simulink model "b_2x_8a_r308d"  (Simulink 6.2)
settings: Solver=ode45  StartTime=0.0  StopTime=1030.0  RelTol=1e-3
undefined symbols (not defined in the file): ant_bits, BEE2_usr, blockCountBits, blockRowBits, cmult_4bit_em
libraries: xbsIndex_r3 x3300, xps_library x102, casper_library x97
(part 5 of 22)

== system b_2x_8a_r308d/snap_gbe_tx ==
  data_in : Inport  Port=1  LatchInput=off
  oob_in : Inport  Port=2  LatchInput=off
  trig : Inport  Port=3  LatchInput=off
  we : Inport  Port=4  LatchInput=off
  Constant : xbsIndex_r3/Constant  const=1  equ=P=C  arith_type=Boolean  n_bits=1  bin_pt=0  opselect=C  inp2=PCIN>>17  opr=+  inp1=P  carry=CIN  iostate=0  explicit_period=on  period=1  dbl_ovrd=off
  Constant1 : xbsIndex_r3/Constant  const=1  equ=P=C  arith_type=Boolean  n_bits=1  bin_pt=0  opselect=C  inp2=PCIN>>17  opr=+  inp1=P  carry=CIN  iostate=0  explicit_period=on  period=1  dbl_ovrd=off
  Constant13 : Constant
  Constant2 : xbsIndex_r3/Constant  const=1  equ=P=C  arith_type=Boolean  n_bits=1  bin_pt=0  opselect=C  inp2=PCIN>>17  opr=+  inp1=P  carry=CIN  iostate=0  explicit_period=on  period=1  dbl_ovrd=off
  Inverter : xbsIndex_r3/Inverter  latency=0  explicit_period=off  period=1  en=off  dbl_ovrd=off  show_param=off
      settings: xl_area=[0, 0, 0, 0, 0, 0, 0]
  Logical1 : xbsIndex_r3/Logical  logical_function=AND  inputs=2  precision=Full  arith_type=Unsigned  n_bits=8  bin_pt=2  align_bp=on  latency=0  explicit_period=off  period=1  en=off  dbl_ovrd=off  show_param=off
      settings: xl_area=[0, 0, 0, 0, 0, 0, 0]
  Mux1 : xbsIndex_r3/Mux  inputs=2  precision=Full  arith_type="Signed  (2's comp)"  n_bits=8  bin_pt=2  quantization=Truncate  overflow=Wrap  latency=0  explicit_period=off  period=1  en=off  dbl_ovrd=off  show_param=off  mux_type=off  use_rpm=off  gen_core=off
      settings: xl_area=[0, 0, 0, 0, 0, 0, 0]
  Mux2 : xbsIndex_r3/Mux  inputs=2  precision=Full  arith_type="Signed  (2's comp)"  n_bits=8  bin_pt=2  quantization=Truncate  overflow=Wrap  latency=0  explicit_period=off  period=1  en=off  dbl_ovrd=off  show_param=off  mux_type=off  use_rpm=off  gen_core=off
      settings: xl_area=[0, 0, 0, 0, 0, 0, 0]
  Register : xbsIndex_r3/Register  init=0  reg_only_valid=off  explicit_period=off  period=1  rst=on  en=on  out_en=off  dbl_ovrd=off  show_param=off
      settings: xl_area=[0, 0, 0, 0, 0, 0, 0]
  Register1 : xbsIndex_r3/Register  init=0  reg_only_valid=off  explicit_period=off  period=1  rst=on  en=on  out_en=off  dbl_ovrd=off  show_param=off
      settings: xl_area=[0, 0, 0, 0, 0, 0, 0]
  Reinterpret3 : xbsIndex_r3/Reinterpret  force_arith_type=on  arith_type=Unsigned  force_bin_pt=on  bin_pt=0  force_valid=on
  addr : xps_library/software register  Tag=xps:sw_reg  io_dir=To Processor  arith_type=Unsigned  bitwidth=32  bin_pt=0  sample_period=1  gw_name=b_2x_8a_r308d_snap_gbe_tx_addr_user_data_in
  bram_lsb : xps_library/Shared BRAM  Tag=xps:bram  arith_type=Unsigned  addr_width=nsamples  data_width=32  data_bin_pt=0  init_vals=0  sample_rate=1
  bram_msb : xps_library/Shared BRAM  Tag=xps:bram  arith_type=Unsigned  addr_width=nsamples  data_width=32  data_bin_pt=0  init_vals=0  sample_rate=1
  bram_oob : xps_library/Shared BRAM  Tag=xps:bram  arith_type=Unsigned  addr_width=nsamples  data_width=32  data_bin_pt=0  init_vals=0  sample_rate=1
  ctrl : xps_library/software register  Tag=xps:sw_reg  io_dir=From Processor  arith_type=Unsigned  bitwidth=32  bin_pt=0  sample_period=1  gw_name=b_2x_8a_r308d_snap_gbe_tx_ctrl_user_data_out
  en1 : xbsIndex_r3/Slice  mode=Lower Bit Location + Width  nbits=32  bit1=0  base1=LSB of Input  bit0=32  base0=LSB of Input  boolean_output=off  explicit_period=off  period=1  dbl_ovrd=off
  en2 : xbsIndex_r3/Slice  mode=Lower Bit Location + Width  nbits=32  bit1=0  base1=LSB of Input  bit0=0  base0=LSB of Input  boolean_output=off  explicit_period=off  period=1  dbl_ovrd=off
  enable : xbsIndex_r3/Slice  mode=Lower Bit Location + Width  nbits=1  bit1=0  base1=LSB of Input  bit0=0  base0=LSB of Input  boolean_output=on  explicit_period=off  period=1  dbl_ovrd=off
  freeze_cntr : casper_library/Misc/freeze_cntr  CounterBits=nsamples
  posedge : casper_library/Misc/posedge  Tag=Rising Edge Detector
  trig1 : xbsIndex_r3/Slice  mode=Lower Bit Location + Width  nbits=1  bit1=0  base1=LSB of Input  bit0=1  base0=LSB of Input  boolean_output=on  explicit_period=off  period=1  dbl_ovrd=off
  valid : xbsIndex_r3/Slice  mode=Lower Bit Location + Width  nbits=1  bit1=0  base1=LSB of Input  bit0=2  base0=LSB of Input  boolean_output=on  explicit_period=off  period=1  dbl_ovrd=off
  wires:
  freeze_cntr/1 -> bram_lsb/1, bram_msb/1, bram_oob/1, Register1/1
  Register/1 -> freeze_cntr/2
  Mux2/1 -> Logical1/1
  Inverter/1 -> Logical1/2
  Logical1/1 -> Register/2
  valid/1 -> Mux1/1
  trig1/1 -> Mux2/1
  Register1/1 -> addr/1
  Constant2/1 -> Mux1/3
  we/1 -> Mux1/2
  Mux1/1 -> freeze_cntr/1
  Constant1/1 -> Mux2/3
  Constant/1 -> Register/1
  posedge/1 -> Inverter/1, Register1/2, Register/3
  ctrl/1 -> trig1/1, valid/1, enable/1
  Constant13/1 -> ctrl/1
  freeze_cntr/2 -> bram_lsb/3, bram_msb/3, bram_oob/3, Register1/3
  enable/1 -> posedge/1
  trig/1 -> Mux2/2
  Reinterpret3/1 -> en1/1, en2/1
  data_in/1 -> Reinterpret3/1
  en1/1 -> bram_msb/2
  en2/1 -> bram_lsb/2
  oob_in/1 -> bram_oob/2

== system b_2x_8a_r308d/snap_rx ==
  data_in : Inport  Port=1  LatchInput=off
  oob_in : Inport  Port=2  LatchInput=off
  trig : Inport  Port=3  LatchInput=off
  we : Inport  Port=4  LatchInput=off
  Constant : xbsIndex_r3/Constant  const=1  equ=P=C  arith_type=Boolean  n_bits=1  bin_pt=0  opselect=C  inp2=PCIN>>17  opr=+  inp1=P  carry=CIN  iostate=0  explicit_period=on  period=1  dbl_ovrd=off
  Constant1 : xbsIndex_r3/Constant  const=1  equ=P=C  arith_type=Boolean  n_bits=1  bin_pt=0  opselect=C  inp2=PCIN>>17  opr=+  inp1=P  carry=CIN  iostate=0  explicit_period=on  period=1  dbl_ovrd=off
  Constant13 : Constant
  Constant2 : xbsIndex_r3/Constant  const=1  equ=P=C  arith_type=Boolean  n_bits=1  bin_pt=0  opselect=C  inp2=PCIN>>17  opr=+  inp1=P  carry=CIN  iostate=0  explicit_period=on  period=1  dbl_ovrd=off
  Inverter : xbsIndex_r3/Inverter  latency=0  explicit_period=off  period=1  en=off  dbl_ovrd=off  show_param=off
      settings: xl_area=[0, 0, 0, 0, 0, 0, 0]
  Logical1 : xbsIndex_r3/Logical  logical_function=AND  inputs=2  precision=Full  arith_type=Unsigned  n_bits=8  bin_pt=2  align_bp=on  latency=0  explicit_period=off  period=1  en=off  dbl_ovrd=off  show_param=off
      settings: xl_area=[0, 0, 0, 0, 0, 0, 0]
  Mux1 : xbsIndex_r3/Mux  inputs=2  precision=Full  arith_type="Signed  (2's comp)"  n_bits=8  bin_pt=2  quantization=Truncate  overflow=Wrap  latency=0  explicit_period=off  period=1  en=off  dbl_ovrd=off  show_param=off  mux_type=off  use_rpm=off  gen_core=off
      settings: xl_area=[0, 0, 0, 0, 0, 0, 0]
  Mux2 : xbsIndex_r3/Mux  inputs=2  precision=Full  arith_type="Signed  (2's comp)"  n_bits=8  bin_pt=2  quantization=Truncate  overflow=Wrap  latency=0  explicit_period=off  period=1  en=off  dbl_ovrd=off  show_param=off  mux_type=off  use_rpm=off  gen_core=off
      settings: xl_area=[0, 0, 0, 0, 0, 0, 0]
  Register : xbsIndex_r3/Register  init=0  reg_only_valid=off  explicit_period=off  period=1  rst=on  en=on  out_en=off  dbl_ovrd=off  show_param=off
      settings: xl_area=[0, 0, 0, 0, 0, 0, 0]
  Register1 : xbsIndex_r3/Register  init=0  reg_only_valid=off  explicit_period=off  period=1  rst=on  en=on  out_en=off  dbl_ovrd=off  show_param=off
      settings: xl_area=[0, 0, 0, 0, 0, 0, 0]
  Reinterpret3 : xbsIndex_r3/Reinterpret  force_arith_type=on  arith_type=Unsigned  force_bin_pt=on  bin_pt=0  force_valid=on
  addr : xps_library/software register  Tag=xps:sw_reg  io_dir=To Processor  arith_type=Unsigned  bitwidth=32  bin_pt=0  sample_period=1  gw_name=b_2x_8a_r308d_snap_rx_addr_user_data_in
  bram_lsb : xps_library/Shared BRAM  Tag=xps:bram  arith_type=Unsigned  addr_width=nsamples  data_width=32  data_bin_pt=0  init_vals=0  sample_rate=1
  bram_msb : xps_library/Shared BRAM  Tag=xps:bram  arith_type=Unsigned  addr_width=nsamples  data_width=32  data_bin_pt=0  init_vals=0  sample_rate=1
  bram_oob : xps_library/Shared BRAM  Tag=xps:bram  arith_type=Unsigned  addr_width=nsamples  data_width=32  data_bin_pt=0  init_vals=0  sample_rate=1
  ctrl : xps_library/software register  Tag=xps:sw_reg  io_dir=From Processor  arith_type=Unsigned  bitwidth=32  bin_pt=0  sample_period=1  gw_name=b_2x_8a_r308d_snap_rx_ctrl_user_data_out
  en1 : xbsIndex_r3/Slice  mode=Lower Bit Location + Width  nbits=32  bit1=0  base1=LSB of Input  bit0=32  base0=LSB of Input  boolean_output=off  explicit_period=off  period=1  dbl_ovrd=off
  en2 : xbsIndex_r3/Slice  mode=Lower Bit Location + Width  nbits=32  bit1=0  base1=LSB of Input  bit0=0  base0=LSB of Input  boolean_output=off  explicit_period=off  period=1  dbl_ovrd=off
  enable : xbsIndex_r3/Slice  mode=Lower Bit Location + Width  nbits=1  bit1=0  base1=LSB of Input  bit0=0  base0=LSB of Input  boolean_output=on  explicit_period=off  period=1  dbl_ovrd=off
  freeze_cntr : casper_library/Misc/freeze_cntr  CounterBits=nsamples
  posedge : casper_library/Misc/posedge  Tag=Rising Edge Detector
  trig1 : xbsIndex_r3/Slice  mode=Lower Bit Location + Width  nbits=1  bit1=0  base1=LSB of Input  bit0=1  base0=LSB of Input  boolean_output=on  explicit_period=off  period=1  dbl_ovrd=off
  valid : xbsIndex_r3/Slice  mode=Lower Bit Location + Width  nbits=1  bit1=0  base1=LSB of Input  bit0=2  base0=LSB of Input  boolean_output=on  explicit_period=off  period=1  dbl_ovrd=off
  wires:
  freeze_cntr/1 -> bram_lsb/1, bram_msb/1, bram_oob/1, Register1/1
  Register/1 -> freeze_cntr/2
  Mux2/1 -> Logical1/1
  Inverter/1 -> Logical1/2
  Logical1/1 -> Register/2
  valid/1 -> Mux1/1
  trig1/1 -> Mux2/1
  Register1/1 -> addr/1
  Constant2/1 -> Mux1/3
  we/1 -> Mux1/2
  Mux1/1 -> freeze_cntr/1
  Constant1/1 -> Mux2/3
  Constant/1 -> Register/1
  posedge/1 -> Inverter/1, Register1/2, Register/3
  ctrl/1 -> trig1/1, valid/1, enable/1
  Constant13/1 -> ctrl/1
  freeze_cntr/2 -> bram_lsb/3, bram_msb/3, bram_oob/3, Register1/3
  enable/1 -> posedge/1
  trig/1 -> Mux2/2
  Reinterpret3/1 -> en1/1, en2/1
  data_in/1 -> Reinterpret3/1
  en1/1 -> bram_msb/2
  en2/1 -> bram_lsb/2
  oob_in/1 -> bram_oob/2

== system b_2x_8a_r308d/snap_xaui ==
  data_in : Inport  Port=1  LatchInput=off
  oob_in : Inport  Port=2  LatchInput=off
  trig : Inport  Port=3  LatchInput=off
  we : Inport  Port=4  LatchInput=off
  Constant : xbsIndex_r3/Constant  const=1  equ=P=C  arith_type=Boolean  n_bits=1  bin_pt=0  opselect=C  inp2=PCIN>>17  opr=+  inp1=P  carry=CIN  iostate=0  explicit_period=on  period=1  dbl_ovrd=off
  Constant1 : xbsIndex_r3/Constant  const=1  equ=P=C  arith_type=Boolean  n_bits=1  bin_pt=0  opselect=C  inp2=PCIN>>17  opr=+  inp1=P  carry=CIN  iostate=0  explicit_period=on  period=1  dbl_ovrd=off
  Constant13 : Constant
  Constant2 : xbsIndex_r3/Constant  const=1  equ=P=C  arith_type=Boolean  n_bits=1  bin_pt=0  opselect=C  inp2=PCIN>>17  opr=+  inp1=P  carry=CIN  iostate=0  explicit_period=on  period=1  dbl_ovrd=off
  Inverter : xbsIndex_r3/Inverter  latency=0  explicit_period=off  period=1  en=off  dbl_ovrd=off  show_param=off
      settings: xl_area=[0, 0, 0, 0, 0, 0, 0]
  Logical1 : xbsIndex_r3/Logical  logical_function=AND  inputs=2  precision=Full  arith_type=Unsigned  n_bits=8  bin_pt=2  align_bp=on  latency=0  explicit_period=off  period=1  en=off  dbl_ovrd=off  show_param=off
      settings: xl_area=[0, 0, 0, 0, 0, 0, 0]
  Mux1 : xbsIndex_r3/Mux  inputs=2  precision=Full  arith_type="Signed  (2's comp)"  n_bits=8  bin_pt=2  quantization=Truncate  overflow=Wrap  latency=0  explicit_period=off  period=1  en=off  dbl_ovrd=off  show_param=off  mux_type=off  use_rpm=off  gen_core=off
      settings: xl_area=[0, 0, 0, 0, 0, 0, 0]
  Mux2 : xbsIndex_r3/Mux  inputs=2  precision=Full  arith_type="Signed  (2's comp)"  n_bits=8  bin_pt=2  quantization=Truncate  overflow=Wrap  latency=0  explicit_period=off  period=1  en=off  dbl_ovrd=off  show_param=off  mux_type=off  use_rpm=off  gen_core=off
      settings: xl_area=[0, 0, 0, 0, 0, 0, 0]
  Register : xbsIndex_r3/Register  init=0  reg_only_valid=off  explicit_period=off  period=1  rst=on  en=on  out_en=off  dbl_ovrd=off  show_param=off
      settings: xl_area=[0, 0, 0, 0, 0, 0, 0]
  Register1 : xbsIndex_r3/Register  init=0  reg_only_valid=off  explicit_period=off  period=1  rst=on  en=on  out_en=off  dbl_ovrd=off  show_param=off
      settings: xl_area=[0, 0, 0, 0, 0, 0, 0]
  Reinterpret3 : xbsIndex_r3/Reinterpret  force_arith_type=on  arith_type=Unsigned  force_bin_pt=on  bin_pt=0  force_valid=on
  addr : xps_library/software register  Tag=xps:sw_reg  io_dir=To Processor  arith_type=Unsigned  bitwidth=32  bin_pt=0  sample_period=1  gw_name=b_2x_8a_r308d_snap_xaui_addr_user_data_in
  bram_lsb : xps_library/Shared BRAM  Tag=xps:bram  arith_type=Unsigned  addr_width=nsamples  data_width=32  data_bin_pt=0  init_vals=0  sample_rate=1
  bram_msb : xps_library/Shared BRAM  Tag=xps:bram  arith_type=Unsigned  addr_width=nsamples  data_width=32  data_bin_pt=0  init_vals=0  sample_rate=1
  bram_oob : xps_library/Shared BRAM  Tag=xps:bram  arith_type=Unsigned  addr_width=nsamples  data_width=32  data_bin_pt=0  init_vals=0  sample_rate=1
  ctrl : xps_library/software register  Tag=xps:sw_reg  io_dir=From Processor  arith_type=Unsigned  bitwidth=32  bin_pt=0  sample_period=1  gw_name=b_2x_8a_r308d_snap_xaui_ctrl_user_data_out
  en1 : xbsIndex_r3/Slice  mode=Lower Bit Location + Width  nbits=32  bit1=0  base1=LSB of Input  bit0=32  base0=LSB of Input  boolean_output=off  explicit_period=off  period=1  dbl_ovrd=off
  en2 : xbsIndex_r3/Slice  mode=Lower Bit Location + Width  nbits=32  bit1=0  base1=LSB of Input  bit0=0  base0=LSB of Input  boolean_output=off  explicit_period=off  period=1  dbl_ovrd=off
  enable : xbsIndex_r3/Slice  mode=Lower Bit Location + Width  nbits=1  bit1=0  base1=LSB of Input  bit0=0  base0=LSB of Input  boolean_output=on  explicit_period=off  period=1  dbl_ovrd=off
  freeze_cntr : casper_library/Misc/freeze_cntr  CounterBits=nsamples
  posedge : casper_library/Misc/posedge  Tag=Rising Edge Detector
  trig1 : xbsIndex_r3/Slice  mode=Lower Bit Location + Width  nbits=1  bit1=0  base1=LSB of Input  bit0=1  base0=LSB of Input  boolean_output=on  explicit_period=off  period=1  dbl_ovrd=off
  valid : xbsIndex_r3/Slice  mode=Lower Bit Location + Width  nbits=1  bit1=0  base1=LSB of Input  bit0=2  base0=LSB of Input  boolean_output=on  explicit_period=off  period=1  dbl_ovrd=off
  wires:
  freeze_cntr/1 -> bram_lsb/1, bram_msb/1, bram_oob/1, Register1/1
  Register/1 -> freeze_cntr/2
  Mux2/1 -> Logical1/1
  Inverter/1 -> Logical1/2
  Logical1/1 -> Register/2
  valid/1 -> Mux1/1
  trig1/1 -> Mux2/1
  Register1/1 -> addr/1
  Constant2/1 -> Mux1/3
  we/1 -> Mux1/2
  Mux1/1 -> freeze_cntr/1
  Constant1/1 -> Mux2/3
  Constant/1 -> Register/1
  posedge/1 -> Inverter/1, Register1/2, Register/3
  ctrl/1 -> trig1/1, valid/1, enable/1
  Constant13/1 -> ctrl/1
  freeze_cntr/2 -> bram_lsb/3, bram_msb/3, bram_oob/3, Register1/3
  enable/1 -> posedge/1
  trig/1 -> Mux2/2
  Reinterpret3/1 -> en1/1, en2/1
  data_in/1 -> Reinterpret3/1
  en1/1 -> bram_msb/2
  en2/1 -> bram_lsb/2
  oob_in/1 -> bram_oob/2

== system b_2x_8a_r308d/snap_xout1 ==
  note: could not route with
      | brams size2^14
  data_in : Inport  Port=1  LatchInput=off
  valid_in : Inport  Port=2  LatchInput=off
  trigger : Inport  Port=3  LatchInput=off
  reset : Inport  Port=4  LatchInput=off
  1 : xbsIndex_r3/Slice  mode=Lower Bit Location + Width  nbits=32  bit1=0  base1=LSB of Input  bit0=96  base0=LSB of Input  boolean_output=on  explicit_period=off  period=1  dbl_ovrd=off
  2 : xbsIndex_r3/Slice  mode=Lower Bit Location + Width  nbits=32  bit1=0  base1=LSB of Input  bit0=64  base0=LSB of Input  boolean_output=on  explicit_period=off  period=1  dbl_ovrd=off
  3 : xbsIndex_r3/Slice  mode=Lower Bit Location + Width  nbits=32  bit1=0  base1=LSB of Input  bit0=32  base0=LSB of Input  boolean_output=on  explicit_period=off  period=1  dbl_ovrd=off
  4 : xbsIndex_r3/Slice  mode=Lower Bit Location + Width  nbits=32  bit1=0  base1=LSB of Input  bit0=0  base0=LSB of Input  boolean_output=on  explicit_period=off  period=1  dbl_ovrd=off
  Constant : xbsIndex_r3/Constant  const=1  equ=P=C  arith_type=Boolean  n_bits=1  bin_pt=0  opselect=C  inp2=PCIN>>17  opr=+  inp1=P  carry=CIN  iostate=0  explicit_period=on  period=1  dbl_ovrd=off
  Gateway Out{1..3,13..15} (6 alike) : xbsIndex_r3/Gateway Out  output_type=Double  nbits=8  bin_pt=6  arith_type=Boolean  quantization=Truncate  overflow=Wrap  hdl_port=off  timing_constraint=None  locs_specified=off  LOCs={}  needs_fixed_name=off  show_param=off
      settings: xl_area=[0, 0, 0, 0, 0, 0, 0]
  Inverter1 : xbsIndex_r3/Inverter  latency=0  explicit_period=off  period=1  en=off  dbl_ovrd=off  show_param=off
      settings: xl_area=[0, 0, 0, 0, 0, 0, 0]
  Logical5 : xbsIndex_r3/Logical  logical_function=AND  inputs=2  precision=Full  arith_type=Unsigned  n_bits=8  bin_pt=2  align_bp=on  latency=0  explicit_period=off  period=1  en=off  dbl_ovrd=off  show_param=off
      settings: xl_area=[0, 0, 0, 0, 0, 0, 0]
  Register : xbsIndex_r3/Register  init=0  reg_only_valid=off  explicit_period=off  period=1  rst=on  en=on  out_en=off  dbl_ovrd=off  show_param=off
      settings: xl_area=[0, 0, 0, 0, 0, 0, 0]
  Register2 : xbsIndex_r3/Register  init=0  reg_only_valid=off  explicit_period=off  period=1  rst=on  en=on  out_en=off  dbl_ovrd=off  show_param=off
      settings: xl_area=[0, 0, 0, 0, 0, 0, 0]
  Scope1 : Scope  NumInputPorts=6
      settings: YMin=272014000~0~0~-5~-5~-5  YMax=300648000~110~1~5~5~5
  addr : xps_library/software register  Tag=xps:sw_reg  io_dir=To Processor  arith_type=Unsigned  bitwidth=32  bin_pt=0  sample_period=1  gw_name=b_2x_8a_r308d_snap_xout1_addr_user_data_in
  bram{0..3} (4 alike) : xps_library/Shared BRAM  Tag=xps:bram  arith_type=Unsigned  addr_width=13  data_width=32  data_bin_pt=0  init_vals=0  sample_rate=1
  freeze_cntr : casper_library/Misc/freeze_cntr  CounterBits=13
  wires:
  4/1 -> bram0/2, Gateway Out15/1
  3/1 -> bram1/2, Gateway Out2/1
  2/1 -> bram2/2, Gateway Out1/1
  1/1 -> bram3/2, Gateway Out3/1
  Gateway Out2/1 -> Scope1/3
  Gateway Out1/1 -> Scope1/2
  Gateway Out3/1 -> Scope1/1
  Gateway Out15/1 -> Scope1/4
  Gateway Out13/1 -> Scope1/5
  Gateway Out14/1 -> Scope1/6
  data_in/1 -> 4/1, 3/1, 2/1, 1/1
  freeze_cntr/1 -> bram0/1, bram1/1, bram2/1, bram3/1, Gateway Out13/1, Register2/1
  Register/1 -> freeze_cntr/2
  freeze_cntr/2 -> Register2/3, bram0/3, bram1/3, bram2/3, bram3/3, Gateway Out14/1
  Constant/1 -> Register/1
  Register2/1 -> addr/1
  Logical5/1 -> Register/2
  Inverter1/1 -> Logical5/2
  reset/1 -> Register2/2, Register/3, Inverter1/1
  valid_in/1 -> freeze_cntr/1
  trigger/1 -> Logical5/1

== system b_2x_8a_r308d/win_x_engine1 ==
  ant : Inport  Port=1  LatchInput=off
  sync_in : Inport  Port=2  LatchInput=off
  window_valid : Inport  Port=3  LatchInput=off
  Constant : xbsIndex_r3/Constant  const=0  equ=P=C  arith_type=Unsigned  n_bits=8 * n_bits_out  bin_pt=0  opselect=C  inp2=PCIN>>17  opr=+  inp1=P  carry=CIN  iostate=0  explicit_period=on  period=1  dbl_ovrd=off
  Constant1 : xbsIndex_r3/Constant  const=0  equ=P=C  arith_type=Boolean  n_bits=1  bin_pt=0  opselect=C  inp2=PCIN>>17  opr=+  inp1=P  carry=CIN  iostate=0  explicit_period=on  period=1  dbl_ovrd=off
  Logical : xbsIndex_r3/Logical  logical_function=AND  inputs=2  precision=Full  arith_type=Unsigned  n_bits=8  bin_pt=2  align_bp=on  latency=0  explicit_period=off  period=1  en=off  dbl_ovrd=off  show_param=off
      settings: xl_area=[0, 0, 0, 0, 0, 0, 0]
  Term1 : Terminator
  Term2 : Terminator
  Term3 : Terminator
  auto_tap : Subsystem  mask(auto_tap){use_ded_mult=1}
      mask prompts: use_ded_mult "Use Dedicated Multipliers"
      mask init:
      | auto_tap_init(gcb, ...
      |     'use_ded_mult', use_ded_mult);
      settings: AttributesFormatString=mult=1
  baseline_tap1 : casper_library/Correlator/baseline_tap  ant_sep=1  use_ded_mult=1  use_bram_delay=1
      link override Constant: equ=P=C
      link override delay/delay_bram/Constant2: equ=P=C
      settings: AttributesFormatString=ant_sep=1, mult=1, bram=1
  baseline_tap2 : Subsystem  AncestorBlock=casper_library/Correlator/baseline_tap  mask(baseline_tap){ant_sep=2, use_ded_mult=1, use_bram_delay=1}
      mask prompts: ant_sep "Antenna Seperation"; use_ded_mult "Multiplier Type (0=slices 1=embedded 2=bram)"; use_bram_delay "Delay in BRAM"
      mask init:
      | baseline_tap_init(gcb, ...
      |     'ant_sep', ant_sep, ...
      |     'use_ded_mult', use_ded_mult, ...
      |     'use_bram_delay', use_bram_delay);
      settings: AttributesFormatString=ant_sep=2, mult=1, bram=1
  baseline_tap3 : Subsystem  AncestorBlock=casper_library/Correlator/baseline_tap  mask(baseline_tap){ant_sep=3, use_ded_mult=1, use_bram_delay=1}
      mask prompts: ant_sep "Antenna Seperation"; use_ded_mult "Multiplier Type (0=slices 1=embedded 2=bram)"; use_bram_delay "Delay in BRAM"
      mask init:
      | baseline_tap_init(gcb, ...
      |     'ant_sep', ant_sep, ...
      |     'use_ded_mult', use_ded_mult, ...
      |     'use_bram_delay', use_bram_delay);
      settings: AttributesFormatString=ant_sep=3, mult=1, bram=1
  baseline_tap4 : Subsystem  AncestorBlock=casper_library/Correlator/baseline_tap  mask(baseline_tap){ant_sep=4, use_ded_mult=1, use_bram_delay=1}
      mask prompts: ant_sep "Antenna Seperation"; use_ded_mult "Multiplier Type (0=slices 1=embedded 2=bram)"; use_bram_delay "Delay in BRAM"
      mask init:
      | baseline_tap_init(gcb, ...
      |     'ant_sep', ant_sep, ...
      |     'use_ded_mult', use_ded_mult, ...
      |     'use_bram_delay', use_bram_delay);
      settings: AttributesFormatString=ant_sep=4, mult=1, bram=1
  window_delay : Subsystem  mask{delay=add_latency + mult_latency + acc_len + floor(n_ants/2 + 1) + 1}
      mask prompts: delay "desired delay (>2)"
      mask Display: fprintf('Z^-%d', delay)
  x_engine_reorder : Subsystem  AncestorBlock=casper_library/Correlator/x_engine_reorder  mask{num_ants=n_ants}
      mask prompts: num_ants "Number of Antennas"
      mask init:
      | num_taps = floor(num_ants/2) + 1;
      | num_validins = num_ants*num_taps;
      | 
      | addr_offset = floor(num_ants/2) * num_taps - sum(1:num_taps-1) - 1;
      | if (mod(num_ants, 2) == 0)
      |     addr_offset = addr_offset - floor(num_ants/2);
      | end
      | 
      | num_elements = nchoosek(num_ants, 2) + num_ants;
      | elements_bits = floor(log2(num_elements)) + 1;
      | 
      | fmtstr = sprintf('num_ants=%d',num_ants);
      | set_param(gcb, 'AttributesFormatString', fmtstr);
      settings: AttributesFormatString=num_ants=8
  acc : Outport
  valid : Outport  Port=2
  sync_out : Outport  Port=3
  wires:
  ant/1 -> auto_tap/1(a_del), auto_tap/2(a_ndel)
  Constant/1 -> auto_tap/4(acc_in)
  Constant1/1 -> auto_tap/5(valid_in)
  sync_in/1 -> auto_tap/6(sync_in)
  window_valid/1 -> window_delay/1(in)
  window_delay/1(out) -> Logical/2
  Logical/1 -> x_engine_reorder/2(valid)
  x_engine_reorder/1(acc_out) -> acc/1
  x_engine_reorder/2(valid_out) -> valid/1
  x_engine_reorder/3(sync_out) -> sync_out/1
  auto_tap/1(a_del_out) -> baseline_tap1/1
  auto_tap/2(a_ndel_out) -> baseline_tap1/2
  auto_tap/3(a_end_out) -> baseline_tap1/3
  auto_tap/4(acc_out) -> baseline_tap1/4
  auto_tap/5(valid_out) -> baseline_tap1/5
  auto_tap/6(rst_out) -> baseline_tap1/6
  auto_tap/7(sync_out) -> baseline_tap1/7
  baseline_tap1/1 -> baseline_tap2/1(a_del)
  baseline_tap1/2 -> baseline_tap2/2(a_ndel)
  baseline_tap1/3 -> baseline_tap2/3(a_end)
  baseline_tap1/4 -> baseline_tap2/4(acc_in)
  baseline_tap1/5 -> baseline_tap2/5(valid_in)
  baseline_tap1/6 -> baseline_tap2/6(rst)
  baseline_tap1/7 -> baseline_tap2/7(sync1)
  baseline_tap2/1(a_del_out) -> baseline_tap3/1(a_del)
  baseline_tap2/2(a_ndel_out) -> baseline_tap3/2(a_ndel)
  baseline_tap2/3(a_end_out) -> baseline_tap3/3(a_end)
  baseline_tap2/4(acc_out) -> baseline_tap3/4(acc_in)
  baseline_tap2/5(valid_out) -> baseline_tap3/5(valid_in)
  baseline_tap2/6(rst_out) -> baseline_tap3/6(rst)
  baseline_tap2/7(sync_out) -> baseline_tap3/7(sync1)
  baseline_tap3/1(a_del_out) -> baseline_tap4/1(a_del)
  baseline_tap3/2(a_ndel_out) -> baseline_tap4/2(a_ndel)
  baseline_tap3/3(a_end_out) -> baseline_tap4/3(a_end)
  baseline_tap3/4(acc_out) -> baseline_tap4/4(acc_in)
  baseline_tap3/5(valid_out) -> baseline_tap4/5(valid_in)
  baseline_tap3/6(rst_out) -> baseline_tap4/6(rst)
  baseline_tap3/7(sync_out) -> baseline_tap4/7(sync1)
  baseline_tap4/1(a_del_out) -> auto_tap/3(a_loop)
  baseline_tap4/2(a_ndel_out) -> Term1/1
  baseline_tap4/3(a_end_out) -> Term2/1
  baseline_tap4/4(acc_out) -> x_engine_reorder/1(acc)
  baseline_tap4/5(valid_out) -> Logical/1
  baseline_tap4/6(rst_out) -> Term3/1
  baseline_tap4/7(sync_out) -> x_engine_reorder/3(sync)

== system b_2x_8a_r308d/win_x_engine2 ==
  ant : Inport  Port=1  LatchInput=off
  sync_in : Inport  Port=2  LatchInput=off
  window_valid : Inport  Port=3  LatchInput=off
  Constant : xbsIndex_r3/Constant  const=0  equ=P=C  arith_type=Unsigned  n_bits=8 * n_bits_out  bin_pt=0  opselect=C  inp2=PCIN>>17  opr=+  inp1=P  carry=CIN  iostate=0  explicit_period=on  period=1  dbl_ovrd=off
  Constant1 : xbsIndex_r3/Constant  const=0  equ=P=C  arith_type=Boolean  n_bits=1  bin_pt=0  opselect=C  inp2=PCIN>>17  opr=+  inp1=P  carry=CIN  iostate=0  explicit_period=on  period=1  dbl_ovrd=off
  Logical : xbsIndex_r3/Logical  logical_function=AND  inputs=2  precision=Full  arith_type=Unsigned  n_bits=8  bin_pt=2  align_bp=on  latency=0  explicit_period=off  period=1  en=off  dbl_ovrd=off  show_param=off
      settings: xl_area=[0, 0, 0, 0, 0, 0, 0]
  Term1 : Terminator
  Term2 : Terminator
  Term3 : Terminator
  auto_tap : Subsystem  mask(auto_tap){use_ded_mult=1}
      mask prompts: use_ded_mult "Use Dedicated Multipliers"
      mask init:
      | auto_tap_init(gcb, ...
      |     'use_ded_mult', use_ded_mult);
      settings: AttributesFormatString=mult=1
  baseline_tap1 : casper_library/Correlator/baseline_tap  ant_sep=1  use_ded_mult=1  use_bram_delay=1
      link override Constant: equ=P=C
      link override delay/delay_bram/Constant2: equ=P=C
      settings: AttributesFormatString=ant_sep=1, mult=1, bram=1
  baseline_tap2 : Subsystem  AncestorBlock=casper_library/Correlator/baseline_tap  mask(baseline_tap){ant_sep=2, use_ded_mult=1, use_bram_delay=1}
      mask prompts: ant_sep "Antenna Seperation"; use_ded_mult "Multiplier Type (0=slices 1=embedded 2=bram)"; use_bram_delay "Delay in BRAM"
      mask init:
      | baseline_tap_init(gcb, ...
      |     'ant_sep', ant_sep, ...
      |     'use_ded_mult', use_ded_mult, ...
      |     'use_bram_delay', use_bram_delay);
      settings: AttributesFormatString=ant_sep=2, mult=1, bram=1
  baseline_tap3 : Subsystem  AncestorBlock=casper_library/Correlator/baseline_tap  mask(baseline_tap){ant_sep=3, use_ded_mult=1, use_bram_delay=1}
      mask prompts: ant_sep "Antenna Seperation"; use_ded_mult "Multiplier Type (0=slices 1=embedded 2=bram)"; use_bram_delay "Delay in BRAM"
      mask init:
      | baseline_tap_init(gcb, ...
      |     'ant_sep', ant_sep, ...
      |     'use_ded_mult', use_ded_mult, ...
      |     'use_bram_delay', use_bram_delay);
      settings: AttributesFormatString=ant_sep=3, mult=1, bram=1
  baseline_tap4 : Subsystem  AncestorBlock=casper_library/Correlator/baseline_tap  mask(baseline_tap){ant_sep=4, use_ded_mult=1, use_bram_delay=1}
      mask prompts: ant_sep "Antenna Seperation"; use_ded_mult "Multiplier Type (0=slices 1=embedded 2=bram)"; use_bram_delay "Delay in BRAM"
      mask init:
      | baseline_tap_init(gcb, ...
      |     'ant_sep', ant_sep, ...
      |     'use_ded_mult', use_ded_mult, ...
      |     'use_bram_delay', use_bram_delay);
      settings: AttributesFormatString=ant_sep=4, mult=1, bram=1
  window_delay : Subsystem  mask{delay=add_latency + mult_latency + acc_len + floor(n_ants/2 + 1) + 1}
      mask prompts: delay "desired delay (>2)"
      mask Display: fprintf('Z^-%d', delay)
  x_engine_reorder : Subsystem  AncestorBlock=casper_library/Correlator/x_engine_reorder  mask{num_ants=n_ants}
      mask prompts: num_ants "Number of Antennas"
      mask init: same as b_2x_8a_r308d/win_x_engine1/x_engine_reorder
      settings: AttributesFormatString=num_ants=8
  acc : Outport
  valid : Outport  Port=2
  sync_out : Outport  Port=3
  wires:
  ant/1 -> auto_tap/1(a_del), auto_tap/2(a_ndel)
  Constant/1 -> auto_tap/4(acc_in)
  Constant1/1 -> auto_tap/5(valid_in)
  sync_in/1 -> auto_tap/6(sync_in)
  window_valid/1 -> window_delay/1(in)
  window_delay/1(out) -> Logical/2
  Logical/1 -> x_engine_reorder/2(valid)
  x_engine_reorder/1(acc_out) -> acc/1
  x_engine_reorder/2(valid_out) -> valid/1
  x_engine_reorder/3(sync_out) -> sync_out/1
  auto_tap/1(a_del_out) -> baseline_tap1/1
  auto_tap/2(a_ndel_out) -> baseline_tap1/2
  auto_tap/3(a_end_out) -> baseline_tap1/3
  auto_tap/4(acc_out) -> baseline_tap1/4
  auto_tap/5(valid_out) -> baseline_tap1/5
  auto_tap/6(rst_out) -> baseline_tap1/6
  auto_tap/7(sync_out) -> baseline_tap1/7
  baseline_tap1/1 -> baseline_tap2/1(a_del)
  baseline_tap1/2 -> baseline_tap2/2(a_ndel)
  baseline_tap1/3 -> baseline_tap2/3(a_end)
  baseline_tap1/4 -> baseline_tap2/4(acc_in)
  baseline_tap1/5 -> baseline_tap2/5(valid_in)
  baseline_tap1/6 -> baseline_tap2/6(rst)
  baseline_tap1/7 -> baseline_tap2/7(sync1)
  baseline_tap2/1(a_del_out) -> baseline_tap3/1(a_del)
  baseline_tap2/2(a_ndel_out) -> baseline_tap3/2(a_ndel)
  baseline_tap2/3(a_end_out) -> baseline_tap3/3(a_end)
  baseline_tap2/4(acc_out) -> baseline_tap3/4(acc_in)
  baseline_tap2/5(valid_out) -> baseline_tap3/5(valid_in)
  baseline_tap2/6(rst_out) -> baseline_tap3/6(rst)
  baseline_tap2/7(sync_out) -> baseline_tap3/7(sync1)
  baseline_tap3/1(a_del_out) -> baseline_tap4/1(a_del)
  baseline_tap3/2(a_ndel_out) -> baseline_tap4/2(a_ndel)
  baseline_tap3/3(a_end_out) -> baseline_tap4/3(a_end)
  baseline_tap3/4(acc_out) -> baseline_tap4/4(acc_in)
  baseline_tap3/5(valid_out) -> baseline_tap4/5(valid_in)
  baseline_tap3/6(rst_out) -> baseline_tap4/6(rst)
  baseline_tap3/7(sync_out) -> baseline_tap4/7(sync1)
  baseline_tap4/1(a_del_out) -> auto_tap/3(a_loop)
  baseline_tap4/2(a_ndel_out) -> Term1/1
  baseline_tap4/3(a_end_out) -> Term2/1
  baseline_tap4/4(acc_out) -> x_engine_reorder/1(acc)
  baseline_tap4/5(valid_out) -> Logical/1
  baseline_tap4/6(rst_out) -> Term3/1
  baseline_tap4/7(sync_out) -> x_engine_reorder/3(sync)

== system b_2x_8a_r308d/descramble_window1/deflagger ==
  din : Inport  Port=1  LatchInput=off
  Slice1 : xbsIndex_r3/Slice  mode=Lower Bit Location + Width  nbits=16  bit1=0  base1=MSB of Input  bit0=0  base0=LSB of Input  boolean_output=off  explicit_period=off  period=1  dbl_ovrd=off
  Slice2 : xbsIndex_r3/Slice  mode=Upper Bit Location + Width  nbits=1  bit1=-1  base1=MSB of Input  bit0=0  base0=LSB of Input  boolean_output=on  explicit_period=off  period=1  dbl_ovrd=off
  Slice3 : xbsIndex_r3/Slice  mode=Upper Bit Location + Width  nbits=1  bit1=0  base1=MSB of Input  bit0=0  base0=LSB of Input  boolean_output=on  explicit_period=off  period=1  dbl_ovrd=off
  dout : Outport
  flag : Outport  Port=2
  rcvd : Outport  Port=3
  wires:
  Slice1/1 -> dout/1
  Slice3/1 -> rcvd/1
  Slice2/1 -> flag/1
  din/1 -> Slice3/1, Slice2/1, Slice1/1

== system b_2x_8a_r308d/descramble_window1/flagger ==
  flag : Inport  Port=1  LatchInput=off
  din : Inport  Port=2  LatchInput=off
  Concat : xbsIndex_r3/Concat  num_inputs=12  explicit_period=off  period=1  dbl_ovrd=off
  Constant{1..4} (4 alike) : xbsIndex_r3/Constant  const=1  equ=P=C  arith_type=Unsigned  n_bits=1  bin_pt=0  opselect=C  inp2=PCIN>>17  opr=+  inp1=P  carry=CIN  iostate=0  explicit_period=on  period=1  dbl_ovrd=off
  Slice1 : xbsIndex_r3/Slice  mode=Lower Bit Location + Width  nbits=16  bit1=0  base1=MSB of Input  bit0=0  base0=LSB of Input  boolean_output=off  explicit_period=off  period=1  dbl_ovrd=off
  Slice2 : xbsIndex_r3/Slice  mode=Lower Bit Location + Width  nbits=16  bit1=0  base1=MSB of Input  bit0=16  base0=LSB of Input  boolean_output=off  explicit_period=off  period=1  dbl_ovrd=off
  Slice3 : xbsIndex_r3/Slice  mode=Lower Bit Location + Width  nbits=16  bit1=0  base1=MSB of Input  bit0=32  base0=LSB of Input  boolean_output=off  explicit_period=off  period=1  dbl_ovrd=off
  Slice4 : xbsIndex_r3/Slice  mode=Lower Bit Location + Width  nbits=16  bit1=0  base1=MSB of Input  bit0=48  base0=LSB of Input  boolean_output=off  explicit_period=off  period=1  dbl_ovrd=off
  dout : Outport
  wires:
  Concat/1 -> dout/1
  din/1 -> Slice4/1, Slice3/1, Slice2/1, Slice1/1
  flag/1 -> Concat/11, Concat/8, Concat/5, Concat/2
  Slice4/1 -> Concat/12
  Slice3/1 -> Concat/9
  Slice2/1 -> Concat/6
  Slice1/1 -> Concat/3
  Constant1/1 -> Concat/10
  Constant2/1 -> Concat/7
  Constant3/1 -> Concat/4
  Constant4/1 -> Concat/1

== system b_2x_8a_r308d/descramble_window1/window_addr_gen ==
  note: one extra delay
      | here to align sync
  note: If reading from addr 0 (corresponding to f=0,nant,2nant,...)
      | and max_mcnt (skipping window_bits for the difference
      | between max_mcnt and rd_mcnt) is 0 for sync_bits, then
      | issue a sync.
  note: Allow writing to windows
      | up to 1/2 the total buffer size
      |  behind the current maximum mcnt
  note: Count off spectra
      | within a freq,baseline
      | packet.  Counting for
      | 64 bit word = 4 x 16bit samples
  note: Decide of each window
      | edge whether to read
      | out a window of data
  note: If the read window is 1/2
      | the total buffer size (or more)
      | behind the write window,
      | it is time to ship it out.
  note: rd_addr is counting for
      | 16 bit words output to
      | X engines
  note: Disallow writing to high addresses
      | not accepted by mcnt_thresh
  mcnt : Inport  Port=1  LatchInput=off
  ant : Inport  Port=2  LatchInput=off
  eof : Inport  Port=3  LatchInput=off
  valid : Inport  Port=4  LatchInput=off
  AddSub : xbsIndex_r3/AddSub  mode=Addition  precision=User Defined  arith_type=Unsigned  n_bits=48 - ant_bits  bin_pt=0  quantization=Truncate  overflow=Wrap  latency=2  explicit_period=off  period=1  use_carryin=off  use_carryout=off  en=off  dbl_ovrd=off  show_param=off  use_core=on  pipeline=off  use_rpm=on  gen_core=off
      settings: xl_area=[0, 0, 0, 0, 0, 0, 0]
  AddSub1 : xbsIndex_r3/AddSub  mode=Subtraction  precision=User Defined  arith_type=Unsigned  n_bits=window_bits  bin_pt=0  quantization=Truncate  overflow=Wrap  latency=2  explicit_period=off  period=1  use_carryin=off  use_carryout=off  en=off  dbl_ovrd=off  show_param=off  use_core=on  pipeline=off  use_rpm=on  gen_core=off
      settings: xl_area=[0, 0, 0, 0, 0, 0, 0]
  Concat : xbsIndex_r3/Concat  num_inputs=3  explicit_period=off  period=1  dbl_ovrd=off
  Concat1 : xbsIndex_r3/Concat  num_inputs=2  explicit_period=off  period=1  dbl_ovrd=off
  Constant : xbsIndex_r3/Constant  const=2^(window_bits - 1)  equ=P=C  arith_type=Unsigned  n_bits=48 - ant_bits  bin_pt=0  opselect=C  inp2=PCIN>>17  opr=+  inp1=P  carry=CIN  iostate=0  explicit_period=on  period=1  dbl_ovrd=off
  Constant1 : xbsIndex_r3/Constant  const=2^(window_bits - 1)  equ=P=C  arith_type=Unsigned  n_bits=window_bits  bin_pt=0  opselect=C  inp2=PCIN>>17  opr=+  inp1=P  carry=CIN  iostate=0  explicit_period=on  period=1  dbl_ovrd=off
  Constant3 : xbsIndex_r3/Constant  const=0  equ=P=C  arith_type=Unsigned  n_bits=sync_bits - x_int_bits - ant_bits - window_bits  bin_pt=0  opselect=C  inp2=PCIN>>17  opr=+  inp1=P  carry=CIN  iostate=0  explicit_period=on  period=1  dbl_ovrd=off
  Delay1 : xbsIndex_r3/Delay  latency=3  reg_retiming=off  explicit_period=off  period=1  en=off  accept_only_valid=off  init_zero=on  dbl_ovrd=off  show_param=off
      settings: xl_area=[0, 0, 0, 0, 0, 0, 0]
  Delay2 : xbsIndex_r3/Delay  latency=3  reg_retiming=off  explicit_period=off  period=1  en=off  accept_only_valid=off  init_zero=on  dbl_ovrd=off  show_param=off
      settings: xl_area=[0, 0, 0, 0, 0, 0, 0]
  Delay3 : xbsIndex_r3/Delay  latency=2  reg_retiming=off  explicit_period=off  period=1  en=off  accept_only_valid=off  init_zero=on  dbl_ovrd=off  show_param=off
      settings: xl_area=[0, 0, 0, 0, 0, 0, 0]
  Delay{4..8} (5 alike) : xbsIndex_r3/Delay  latency=1  reg_retiming=off  explicit_period=off  period=1  en=off  accept_only_valid=off  init_zero=on  dbl_ovrd=off  show_param=off
      settings: xl_area=[0, 0, 0, 0, 0, 0, 0]
  Logical : xbsIndex_r3/Logical  logical_function=AND  inputs=3  precision=Full  arith_type=Unsigned  n_bits=8  bin_pt=2  align_bp=on  latency=0  explicit_period=off  period=1  en=off  dbl_ovrd=off  show_param=off
      settings: xl_area=[0, 0, 0, 0, 0, 0, 0]
  Logical1 : xbsIndex_r3/Logical  logical_function=AND  inputs=2  precision=Full  arith_type=Unsigned  n_bits=8  bin_pt=2  align_bp=on  latency=0  explicit_period=off  period=1  en=off  dbl_ovrd=off  show_param=off
      settings: xl_area=[0, 0, 0, 0, 0, 0, 0]
  Logical2 : xbsIndex_r3/Logical  logical_function=AND  inputs=2  precision=Full  arith_type=Unsigned  n_bits=8  bin_pt=2  align_bp=on  latency=0  explicit_period=off  period=1  en=off  dbl_ovrd=off  show_param=off
      settings: xl_area=[0, 0, 0, 0, 0, 0, 0]
  Relational : xbsIndex_r3/Relational  mode=a<b  latency=1  explicit_period=off  period=1  en=off  dbl_ovrd=off  show_param=off
      settings: xl_area=[0, 0, 0, 0, 0, 0, 0]
  Relational1 : xbsIndex_r3/Relational  mode=a>=b  latency=1  explicit_period=on  period=1  en=off  dbl_ovrd=off  show_param=off
      settings: xl_area=[0, 0, 0, 0, 0, 0, 0]
  Relational2 : xbsIndex_r3/Relational  mode=a>=b  latency=1  explicit_period=off  period=1  en=off  dbl_ovrd=off  show_param=off
      settings: xl_area=[0, 0, 0, 0, 0, 0, 0]
  Relational4 : xbsIndex_r3/Relational  mode=a=b  latency=1  explicit_period=off  period=1  en=off  dbl_ovrd=off  show_param=off
      settings: xl_area=[0, 0, 0, 0, 0, 0, 0]
  Slice : xbsIndex_r3/Slice  mode=Lower Bit Location + Width  nbits=window_bits  bit1=0  base1=MSB of Input  bit0=0  base0=LSB of Input  boolean_output=off  explicit_period=off  period=1  dbl_ovrd=off
  Slice1 : xbsIndex_r3/Slice  mode=Lower Bit Location + Width  nbits=window_bits  bit1=0  base1=MSB of Input  bit0=0  base0=LSB of Input  boolean_output=off  explicit_period=off  period=1  dbl_ovrd=off
  Slice2 : xbsIndex_r3/Slice  mode=Upper Bit Location + Width  nbits=1  bit1=0  base1=MSB of Input  bit0=0  base0=LSB of Input  boolean_output=on  explicit_period=off  period=1  dbl_ovrd=off
  Slice3 : xbsIndex_r3/Slice  mode=Lower Bit Location + Width  nbits=window_bits  bit1=0  base1=MSB of Input  bit0=0  base0=LSB of Input  boolean_output=off  explicit_period=off  period=1  dbl_ovrd=off
  Slice4 : xbsIndex_r3/Slice  mode=Lower Bit Location + Width  nbits=x_int_bits + ant_bits  bit1=0  base1=MSB of Input  bit0=0  base0=LSB of Input  boolean_output=off  explicit_period=off  period=1  dbl_ovrd=off
  Slice5 : xbsIndex_r3/Slice  mode=Two Bit Locations  nbits=window_bits  bit1=sync_bits - x_int_bits - ant_bits - 1  base1=LSB of Input  bit0=window_bits  base0=LSB of Input  boolean_output=off  explicit_period=off  period=1  dbl_ovrd=off
  Slice6 : xbsIndex_r3/Slice  mode=Upper Bit Location + Width  nbits=1  bit1=0  base1=MSB of Input  bit0=0  base0=LSB of Input  boolean_output=on  explicit_period=off  period=1  dbl_ovrd=off
  edge : casper_library/Misc/edge
  edge1 : casper_library/Misc/edge
  freqs_for_ants : Subsystem
  mcnt_thresh : Subsystem
  pulse_ext : casper_library/Misc/pulse_ext  pulse_len=2^(x_int_bits + ant_bits)
  win_addr_cnt : xbsIndex_r3/Counter  cnt_type=Free Running  n_bits=x_int_bits + ant_bits + 1  bin_pt=0  arith_type=Unsigned  start_count=0  cnt_to=Inf  cnt_by_val=1  operation=Up  explicit_period=off  period=1  load_pin=off  rst=off  en=off  dbl_ovrd=off  show_param=off  use_rpm=on  gen_core=off
      settings: xl_area=[0, 0, 0, 0, 0, 0, 0]
  win_cnt : xbsIndex_r3/Counter  cnt_type=Free Running  n_bits=window_bits + 1  bin_pt=0  arith_type=Unsigned  start_count=0  cnt_to=Inf  cnt_by_val=1  operation=Up  explicit_period=off  period=1  load_pin=off  rst=off  en=on  dbl_ovrd=off  show_param=off  use_rpm=on  gen_core=off
      settings: xl_area=[0, 0, 0, 0, 0, 0, 0]
  wr_addr_cnt : xbsIndex_r3/Counter  cnt_type=Free Running  n_bits=x_int_bits - 2  bin_pt=0  arith_type=Unsigned  start_count=0  cnt_to=Inf  cnt_by_val=1  operation=Up  explicit_period=off  period=1  load_pin=off  rst=on  en=on  dbl_ovrd=off  show_param=off  use_rpm=on  gen_core=off
      settings: xl_area=[0, 0, 0, 0, 0, 0, 0]
  rd_addr : Outport
  re : Outport  Port=2
  wr_addr : Outport  Port=3
  we : Outport  Port=4
  sync_out : Outport  Port=5
  wires:
  pulse_ext/1 -> Delay6/1
  Concat1/1 -> Delay4/1
  Delay7/1 -> Concat1/2
  Slice2/1 -> edge1/1
  Slice1/1 -> Concat1/1, AddSub1/2
  Slice4/1 -> Delay7/1
  freqs_for_ants/1(mcnt_out) -> Delay3/1, mcnt_thresh/1(mcnt), AddSub/1, Slice/1
  edge/1 -> Logical1/1
  Slice6/1 -> edge/1
  win_addr_cnt/1 -> Slice4/1, Slice6/1
  Delay6/1 -> re/1
  Delay4/1 -> rd_addr/1
  Relational1/1 -> Logical1/2
  Logical2/1 -> sync_out/1
  Relational4/1 -> Logical2/2
  Slice5/1 -> Relational4/2
  Constant3/1 -> Relational4/1
  edge1/1 -> Logical2/1
  Delay3/1 -> Relational2/2
  Relational2/1 -> Logical/1
  mcnt_thresh/1(maxcnt) -> Relational2/1, Slice5/1, Slice3/1, Relational/1
  Constant/1 -> AddSub/2
  mcnt/1 -> freqs_for_ants/1(mcnt)
  AddSub/1 -> Relational/2
  Slice/1 -> Concat/1
  freqs_for_ants/2(addr) -> Concat/2
  Concat/1 -> Delay1/1
  Delay1/1 -> wr_addr/1
  ant/1 -> freqs_for_ants/2(ant)
  wr_addr_cnt/1 -> Concat/3
  valid/1 -> Delay8/1
  eof/1 -> Delay5/1
  Relational/1 -> Logical/2
  Logical/1 -> we/1
  Delay2/1 -> Logical/3
  Logical1/1 -> win_cnt/1, pulse_ext/1
  Slice3/1 -> AddSub1/1
  win_cnt/1 -> Slice2/1, Slice1/1
  AddSub1/1 -> Relational1/1
  Constant1/1 -> Relational1/2
  Delay5/1 -> wr_addr_cnt/1
  Delay8/1 -> wr_addr_cnt/2, Delay2/1

== system b_2x_8a_r308d/descramble_window2/deflagger ==
  din : Inport  Port=1  LatchInput=off
  Slice1 : xbsIndex_r3/Slice  mode=Lower Bit Location + Width  nbits=16  bit1=0  base1=MSB of Input  bit0=0  base0=LSB of Input  boolean_output=off  explicit_period=off  period=1  dbl_ovrd=off
  Slice2 : xbsIndex_r3/Slice  mode=Upper Bit Location + Width  nbits=1  bit1=-1  base1=MSB of Input  bit0=0  base0=LSB of Input  boolean_output=on  explicit_period=off  period=1  dbl_ovrd=off
  Slice3 : xbsIndex_r3/Slice  mode=Upper Bit Location + Width  nbits=1  bit1=0  base1=MSB of Input  bit0=0  base0=LSB of Input  boolean_output=on  explicit_period=off  period=1  dbl_ovrd=off
  dout : Outport
  flag : Outport  Port=2
  rcvd : Outport  Port=3
  wires:
  din/1 -> Slice1/1, Slice2/1, Slice3/1
  Slice2/1 -> flag/1
  Slice3/1 -> rcvd/1
  Slice1/1 -> dout/1

== system b_2x_8a_r308d/descramble_window2/flagger ==
  flag : Inport  Port=1  LatchInput=off
  din : Inport  Port=2  LatchInput=off
  Concat : xbsIndex_r3/Concat  num_inputs=12  explicit_period=off  period=1  dbl_ovrd=off
  Constant{1..4} (4 alike) : xbsIndex_r3/Constant  const=1  equ=P=C  arith_type=Unsigned  n_bits=1  bin_pt=0  opselect=C  inp2=PCIN>>17  opr=+  inp1=P  carry=CIN  iostate=0  explicit_period=on  period=1  dbl_ovrd=off
  Slice1 : xbsIndex_r3/Slice  mode=Lower Bit Location + Width  nbits=16  bit1=0  base1=MSB of Input  bit0=0  base0=LSB of Input  boolean_output=off  explicit_period=off  period=1  dbl_ovrd=off
  Slice2 : xbsIndex_r3/Slice  mode=Lower Bit Location + Width  nbits=16  bit1=0  base1=MSB of Input  bit0=16  base0=LSB of Input  boolean_output=off  explicit_period=off  period=1  dbl_ovrd=off
  Slice3 : xbsIndex_r3/Slice  mode=Lower Bit Location + Width  nbits=16  bit1=0  base1=MSB of Input  bit0=32  base0=LSB of Input  boolean_output=off  explicit_period=off  period=1  dbl_ovrd=off
  Slice4 : xbsIndex_r3/Slice  mode=Lower Bit Location + Width  nbits=16  bit1=0  base1=MSB of Input  bit0=48  base0=LSB of Input  boolean_output=off  explicit_period=off  period=1  dbl_ovrd=off
  dout : Outport
  wires:
  Constant4/1 -> Concat/1
  Constant3/1 -> Concat/4
  Constant2/1 -> Concat/7
  Constant1/1 -> Concat/10
  Slice1/1 -> Concat/3
  Slice2/1 -> Concat/6
  Slice3/1 -> Concat/9
  Slice4/1 -> Concat/12
  flag/1 -> Concat/2, Concat/5, Concat/8, Concat/11
  din/1 -> Slice1/1, Slice2/1, Slice3/1, Slice4/1
  Concat/1 -> dout/1
